simulink model "chap4_9sim"  (Simulink 8.1)
settings: Solver=ode45  StartTime=0.0  StopTime=5  FixedStep=0.001  RelTol=1e-3
settings Model: Creator=ljk  LastModifiedBy=liujk  ExtModeTrigMode=oneshot  ExtModeArmWhenConnect=off
settings DataIOCC: LimitDataPoints=off  SignalLoggingName=sigsOut
settings OptimizationCC: BooleanDataType=off
settings DebuggingCC: SaveWithParameterizedLinksMsg=none  SignalResolutionControl=TryResolveAllWithWarning  SolverPrmCheckMsg=none  MultiTaskDSMMsg=warning  MultiTaskCondExecSysMsg=none  StrictBusMsg=None
settings HardwareCC: TargetUnknown=on
settings RTWCC: IncludeERTFirstTime=on

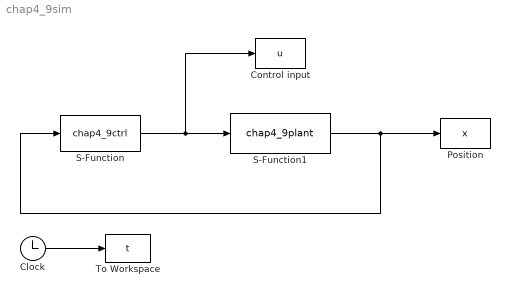
== system chap4_9sim ==
  Clock : Clock
  Control input : ToWorkspace  VariableName=u  SampleTime=-1
  Position : ToWorkspace  VariableName=x  SampleTime=-1
  S-Function : S-Function  FunctionName=chap4_9ctrl  EnableBusSupport=off
  S-Function1 : S-Function  FunctionName=chap4_9plant  EnableBusSupport=off
  To Workspace : ToWorkspace  VariableName=t  SampleTime=-1
  wires:
  S-Function/1 -> S-Function1/1, Control input/1
  S-Function1/1 -> S-Function/1, Position/1
  Clock/1 -> To Workspace/1
